simulink model "Tarea1Parte1SeccionEi"  (R2021a)
settings: Solver=VariableStepAuto  StartTime=0.0  StopTime=10.0  RelTol=1e-3
values from neighbouring files (symbols this model uses):
  K1 = 71.888    [Tarea1Parte1SeccionE.m]    (also in Tarea1_Parte1_Todaslassecciones.m)
  K2 = -10    [Tarea1Parte1SeccionE.m]    (also in Tarea1_Parte1_Todaslassecciones.m)
  Kt = (1/3.3)*100    (= 30.303030303)    [Tarea1Parte1SeccionE.m]    (also in Tarea1_Parte1_Todaslassecciones.m = 0.303; simulink.m)
  Kvc = 0.001    [Tarea1Parte1SeccionE.m]    (also in Tarea1_Parte1_Todaslassecciones.m = 0.1)
  T = 215.664    [Tarea1Parte1SeccionE.m]    (also in Tarea1_Parte1_Todaslassecciones.m)
settings Model: Creator=Royer  LastModifiedBy=Royer

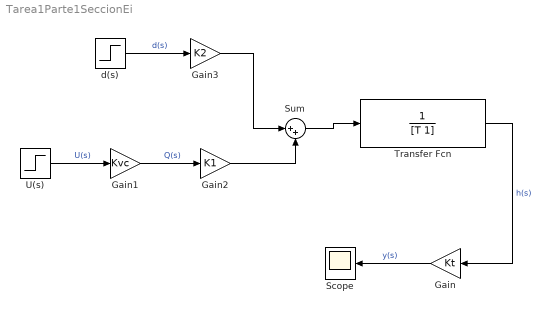
== system Tarea1Parte1SeccionEi ==
  Gain : Gain  Gain=Kt
  Gain1 : Gain  Gain=Kvc
  Gain2 : Gain  Gain=K1
  Gain3 : Gain  Gain=K2
  Scope : Scope
  Sum : Sum  Inputs=|++
  Transfer Fcn : TransferFcn  Denominator=[T 1]
  U(s) : Step  Before=100  SampleTime=0
  d(s) : Step  Before=0.5  SampleTime=0
  wires:
  Transfer Fcn/1 -> Gain/1  "h(s)"
  Gain2/1 -> Sum/2
  Gain1/1 -> Gain2/1  "Q(s)"
  Sum/1 -> Transfer Fcn/1
  Gain/1 -> Scope/1  "y(s)"
  U(s)/1 -> Gain1/1  "U(s)"
  Gain3/1 -> Sum/1
  d(s)/1 -> Gain3/1  "d(s)"
